simulink model "PID"  (R2024a)
settings: Solver=FixedStepAuto  StartTime=0.0  StopTime=inf  RelTol=1e-9  EnableMultiTasking=on
undefined symbols (not defined in the file or in its folder): ln
libraries: arduinolib x2
settings Model: ExtModeTrigDuration=2  Creator=twallema  LastModifiedBy=twallema
settings SolverCC: AlgebraicLoopSolver=TrustRegion
settings OptimizationCC: EnhancedBackFolding=on  PassReuseOutputArgsThreshold=0  MaxStackSize=64  OptimizeBlockOrder=speed  DifferentSizesBufferReuse=on  OptimizationCustomize=off
settings DebuggingCC: ParameterTunabilityLossMsg=error  UnconnectedInputMsg=warning  UnconnectedOutputMsg=warning  UnconnectedLineMsg=warning
settings HardwareCC: ProdBitPerInt=16  ProdBitPerPointer=16  ProdBitPerSizeT=16  ProdBitPerPtrDiffT=16  ProdLargestAtomicFloat=None  ProdWordSize=8  ProdHWDeviceType=Atmel->AVR  UseEmbeddedCoderFeatures=off  UseSimulinkCoderFeatures=off
settings ModelReferenceCC: EnableRefExpFcnMdlSchedulingChecks=on
settings SFSimCC: MATLABDynamicMemAlloc=off  CustomCodeUndefinedFunction=UseInterfaceOnly
settings RTWCC: Description=Embedded Coder  SystemTargetFile=ert.tlc  HardwareBoard=Arduino Uno  TemplateMakefile=ert_default_tmf  GenerateReport=on  Toolchain=Arduino AVR  BuildConfiguration=Faster Runs  LaunchReport=on  GPUComputeCapability=3.5  DLArmComputeVersion=19.05
settings CodeAppCC: ForceParamTrailComments=on  OperatorAnnotations=on
settings ERTTargetCC: ERTCustomFileBanners=off  SupportContinuousTime=on  SupportNonInlinedSFcns=on  RemoveResetFunc=off  SupportVariableSizeSignals=on  ModelStepFunctionPrototypeControlCompliant=off  ExtModeStaticAllocSize=250

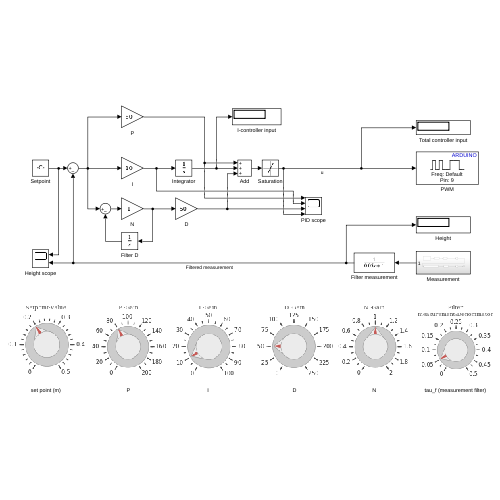
[thumbnail: Simulink's stored preview of the top-level diagram]
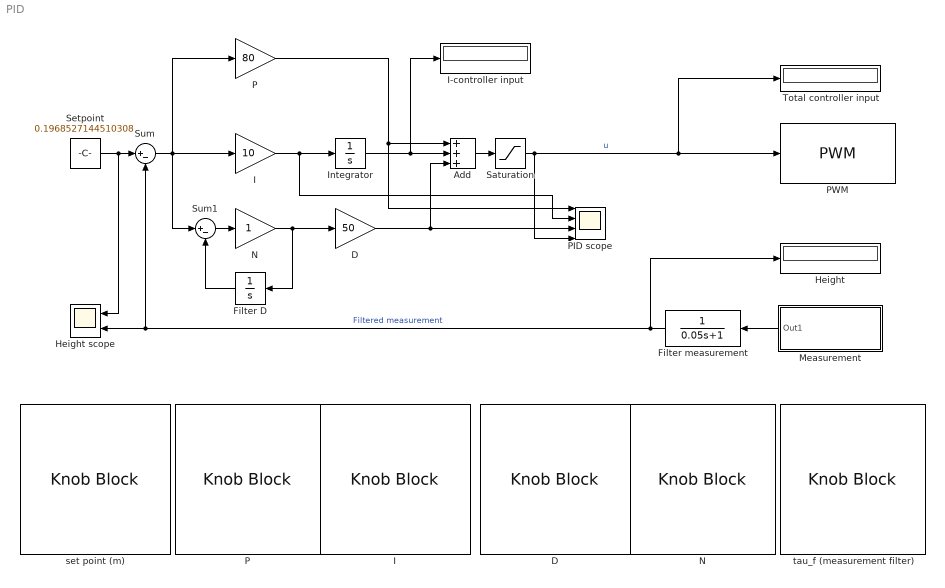
== system PID ==
  Add : Sum  Inputs=+++
  D : KnobBlock  ScaleMax=250
  "D " : Gain  Gain=50
  Filter D : Integrator
  Filter measurement : TransferFcn  Denominator=[0.05,1]
  Height : Display
  Height scope : Scope  NumInputPorts=2
  I : KnobBlock
  "I " : Gain  Gain=10
  I-controller input : Display
  Integrator : Integrator  InitialCondition=151
  Measurement : Subsystem
  N : KnobBlock  ScaleMax=2
  "N " : Gain
  P : KnobBlock  ScaleMax=200
  "P " : Gain  Gain=80
  PID scope : Scope  NumInputPorts=4
  PWM : arduinolib/PWM  pinNumber=9  frequencyType=Default  desiredFrequency=490.2  achievableFrequency=490.2
  Saturation : Saturate  UpperLimit=255  LowerLimit=0
  Setpoint : Constant  Value=0.1968527144510308
  Sum : Sum  Inputs=|+-
  Sum1 : Sum  Inputs=|+-
  Total controller input : Display
  set point (m) : KnobBlock  ScaleMax=0.50  TickInterval=0.1
  tau_f (measurement filter) : KnobBlock  ScaleMax=0.5
  wires:
  Setpoint/1 -> Sum/1, Height scope/1
  Sum/1 -> "P "/1, "I "/1, Sum1/1
  Saturation/1 -> Total controller input/1, PWM/1, PID scope/4  "u"
  Add/1 -> Saturation/1
  "I "/1 -> PID scope/2, Integrator/1
  Integrator/1 -> I-controller input/1, Add/2
  Sum1/1 -> "N "/1
  Filter D/1 -> Sum1/2
  "N "/1 -> Filter D/1, "D "/1
  "D "/1 -> Add/3, PID scope/3
  Filter measurement/1 -> Sum/2, Height scope/2, Height/1  "Filtered measurement"
  "P "/1 -> PID scope/1, Add/1
  Measurement/1(Out1) -> Filter measurement/1

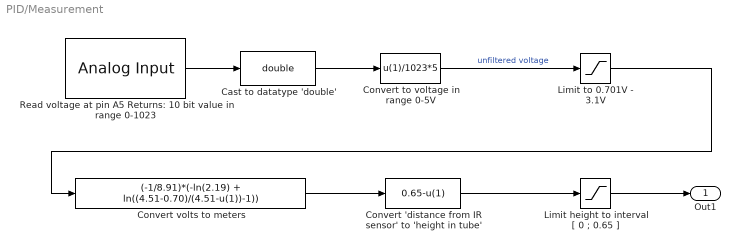
== system PID/Measurement ==
  Cast to datatype 'double' : DataTypeConversion  OutDataTypeStr=double  SaturateOnIntegerOverflow=off  RndMeth=Floor
  Convert 'distance from IR sensor' to 'height in tube' : Fcn  Expr=0.65-u(1)
  Convert to voltage in range 0-5V : Fcn  Expr=u(1)/1023*5
  Convert volts to meters : Fcn  Expr=(-1/8.91)*(-ln(2.19) + ln((4.51-0.70)/(4.51-u(1))-1))
  Limit height to interval [ 0 ; 0.65 ] : Saturate  UpperLimit=0.65  LowerLimit=0
  Limit to 0.701V - 3.1V : Saturate  UpperLimit=3.1  LowerLimit=0.701
  Read voltage at pin A5 Returns: 10 bit value in range 0-1023 : arduinolib/Analog Input  pinNumber=5  ReadResultsOnly=off  ConversionTriggerSource=Software  ExternalTriggerType=uint32(0)  OutputDataType=uint16  EnableConversionCompleteNotify=off  EnableOuputStatus=off  SampleTime=0.1  blockPlatform=arduino
  Out1 : Outport  VectorParamsAs1DForOutWhenUnconnected=off
  wires:
  Convert 'distance from IR sensor' to 'height in tube'/1 -> Limit height to interval [ 0 ; 0.65 ]/1
  Cast to datatype 'double'/1 -> Convert to voltage in range 0-5V/1
  Read voltage at pin A5 Returns: 10 bit value in range 0-1023/1 -> Cast to datatype 'double'/1
  Limit height to interval [ 0 ; 0.65 ]/1 -> Out1/1
  Convert volts to meters/1 -> Convert 'distance from IR sensor' to 'height in tube'/1
  Limit to 0.701V - 3.1V/1 -> Convert volts to meters/1
  Convert to voltage in range 0-5V/1 -> Limit to 0.701V - 3.1V/1  "unfiltered voltage"
